simulink model "Q1b2017"  (R2017b)
settings: Solver=VariableStepAuto  StartTime=0.0  StopTime=100.0  RelTol=1e-3
settings Model: Creator=asus  LastModifiedBy=Kasra
settings CodeAppCC: StateflowObjectComments=on

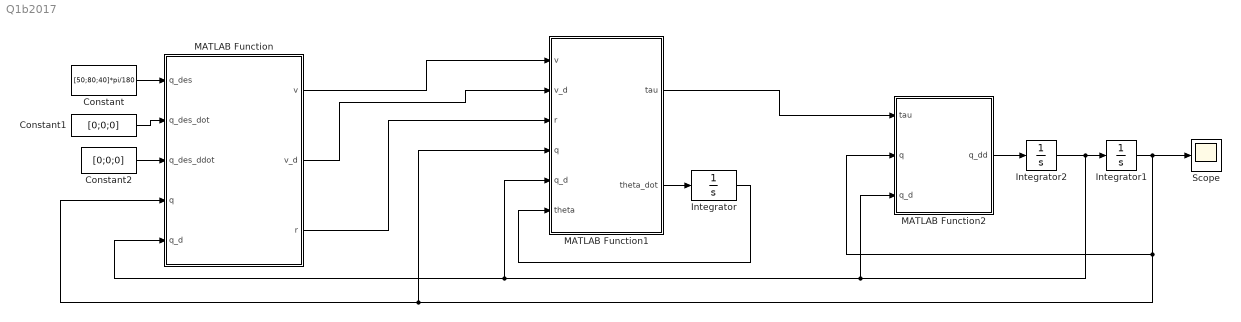
== system Q1b2017 ==
  Constant : Constant  Value=[50;80;40]*pi/180
  Constant1 : Constant  Value=[0;0;0]
  Constant2 : Constant  Value=[0;0;0]
  Integrator : Integrator  InitialCondition=[0;0;0;0]
  Integrator1 : Integrator  InitialCondition=[0;0;0]
  Integrator2 : Integrator  InitialCondition=[0;0;0]
  MATLAB Function : MATLAB Function  TreatAsAtomicUnit=on
  MATLAB Function1 : MATLAB Function  TreatAsAtomicUnit=on
  MATLAB Function2 : MATLAB Function  TreatAsAtomicUnit=on
  Scope : Scope
  wires:
  MATLAB Function/1(v) -> MATLAB Function1/1(v)
  MATLAB Function/2(v_d) -> MATLAB Function1/2(v_d)
  MATLAB Function/3(r) -> MATLAB Function1/3(r)
  MATLAB Function1/2(theta_dot) -> Integrator/1
  Integrator/1 -> MATLAB Function1/6(theta)
  MATLAB Function1/1(tau) -> MATLAB Function2/1(tau)
  MATLAB Function2/1(q_dd) -> Integrator2/1
  Integrator2/1 -> MATLAB Function/5(q_d), MATLAB Function1/5(q_d), MATLAB Function2/3(q_d), Integrator1/1
  Integrator1/1 -> Scope/1, MATLAB Function/4(q), MATLAB Function1/4(q), MATLAB Function2/2(q)
  Constant/1 -> MATLAB Function/1(q_des)
  Constant1/1 -> MATLAB Function/2(q_des_dot)
  Constant2/1 -> MATLAB Function/3(q_des_ddot)

== matlab function Q1b2017/MATLAB Function1 ==
  data: v input; tau output; v_d input; r input; q input; q_d input; theta input; theta_dot output
function [tau,theta_dot]= fcn(v,v_d,r,q,q_d,theta)

g=9.81;
y = [v_d(1), v_d(2), (2*v_d(1)+v_d(2))*cos(q(1))-(q_d(2)*v(2)+q_d(1)*v(2)+v(1)*q_d(2)), 0;0, (v_d(1)+v_d(2)), (v_d(1)*cos(q(2))+(v_d(2)^(2))*sin(q(2))), 0;0, 0, 0, v_d(3)-g];
gam = 0.1;
theta_dot = -pinv(gam)*y'*r;
k = 5*eye(3);
tau = y * theta + k * r;

== matlab function Q1b2017/MATLAB Function ==
  data: q_des input; v output; q_des_dot input; q_des_ddot input; q input; q_d input; v_d output; r output
function [v,v_d,r] = fcn(q_des,q_des_dot,q_des_ddot,q,q_d)
q_tilda = q - q_des;
gamma = 2;
v = q_des_dot - gamma*q_tilda;
q_tilda_dot = q_d - q_des_dot;
v_d = q_des_ddot - gamma * q_tilda_dot;
r = q_d - v;

== matlab function Q1b2017/MATLAB Function2 ==
  data: tau input; q_dd output; q input; q_d input
function q_dd = fcn(tau,q,q_d)

lc1 = 0.3;
lc2 = 0.2;
I1 = 0.36;
I2 = 0.36;
m1=12;
m2=6;
m3=6;
a1 = 0.6;
a2 = 0.4;
g = 9.81;

M11 = m1*lc1^(2)+(m2*(a1^(2)+lc2^(2)+2*a1*lc1*cos(q(2))))+m3*(a1^(2)+a2^(2)+2*a1*a2*cos(q(2)))+I1+I2;
M12 = m2*lc2*(lc2+a1*cos(q(2)))+m3*(a1*a2*cos(q(2))+a2^(2))+I2;
M21 = M12;
M33 = m3;
M22 = m2*lc2^(2)+m3*a2^(2)+I2;
M=[M11, M12, 0;M21, M22, 0;0, 0, M33];
h=(m2*a1*lc2+m3*a2*a1)*sin(q(2));
C=[-2*h*q_d(1), -h*q_d(2), 0;h*q_d(1), 0, 0;0, 0, 0];
G=[0;0;-m3*g];
q_dd = pinv(M)*(tau - C*q_d - G);
